simulink library "linearPlnt_ul"  (R2018a)
settings: Solver=VariableStepAuto  StartTime=0.0  StopTime=10.0  RelTol=1e-3
undefined symbols (not defined in the file): headingTimeConstant_s, maxSteadySpeed_mPs, speedTimeConstant_s
settings Model: Creator=mcobb  LastModifiedBy=mcobb

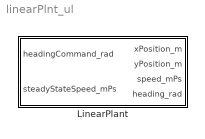
== system linearPlnt_ul ==
  LinearPlant : Subsystem

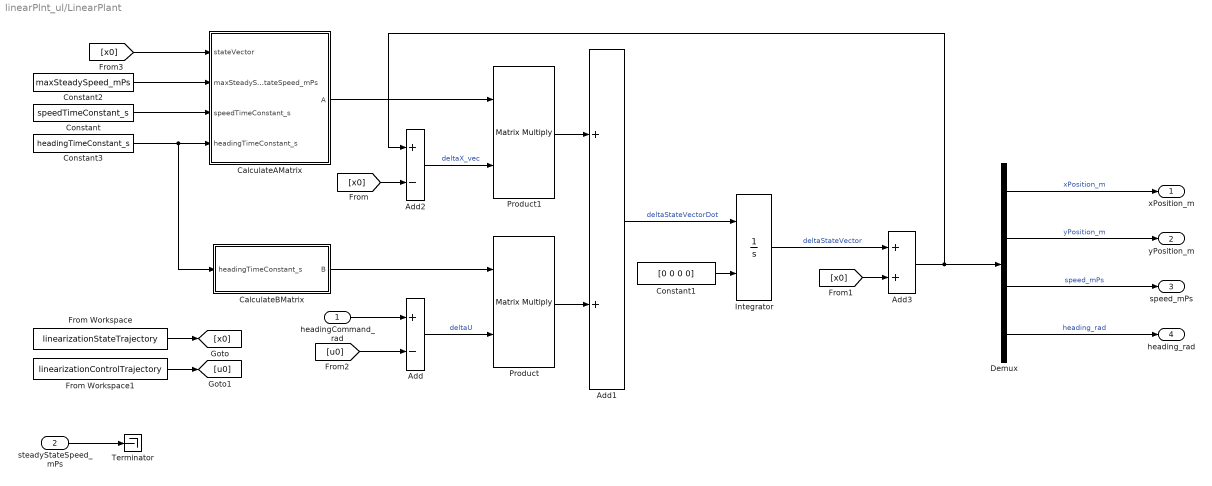
== system linearPlnt_ul/LinearPlant ==
  headingCommand_rad : Inport
  steadyStateSpeed_mPs : Inport  Port=2  PortDimensions=1
  Add : Sum  Inputs=+-
  Add1 : Sum
  Add2 : Sum  Inputs=+-
  Add3 : Sum
  CalculateAMatrix : MATLAB Function  TreatAsAtomicUnit=on
  CalculateBMatrix : MATLAB Function  TreatAsAtomicUnit=on
  Constant : Constant  Value=speedTimeConstant_s
  Constant1 : Constant  Value=[0 0 0 0]
  Constant2 : Constant  Value=maxSteadySpeed_mPs
  Constant3 : Constant  Value=headingTimeConstant_s
  Demux : Demux
  From Workspace : FromWorkspace  VariableName=linearizationStateTrajectory  SampleTime=0
  From Workspace1 : FromWorkspace  VariableName=linearizationControlTrajectory  SampleTime=0
  Integrator : Integrator  InitialConditionSource=external
  Product : Product  Multiplication=Matrix(*)
  Product1 : Product  Multiplication=Matrix(*)
  Terminator : Terminator
  xPosition_m : Outport
  yPosition_m : Outport  Port=2
  speed_mPs : Outport  Port=3
  heading_rad : Outport  Port=4
  wires:
  headingCommand_rad/1 -> Add/1
  Add/1 -> Product/2  "deltaU"
  Product/1 -> Add1/2
  Add2/1 -> Product1/2  "deltaX_vec"
  Add1/1 -> Integrator/1  "deltaStateVectorDot"
  Integrator/1 -> Add3/1  "deltaStateVector"
  Demux/1 -> xPosition_m/1  "xPosition_m"
  Demux/2 -> yPosition_m/1  "yPosition_m"
  Demux/3 -> speed_mPs/1  "speed_mPs"
  Demux/4 -> heading_rad/1  "heading_rad"
  Constant/1 -> CalculateAMatrix/3(speedTimeConstant_s)
  Constant3/1 -> CalculateBMatrix/1(headingTimeConstant_s), CalculateAMatrix/4(headingTimeConstant_s)
  CalculateBMatrix/1(B) -> Product/1
  CalculateAMatrix/1(A) -> Product1/1
  Product1/1 -> Add1/1
  From Workspace/1 -> [x0]
  [x0] -> Add2/2
  Add3/1 -> Add2/1, Demux/1
  [x0] -> Add3/2
  From Workspace1/1 -> [u0]
  [u0] -> Add/2
  Constant1/1 -> Integrator/2
  steadyStateSpeed_mPs/1 -> Terminator/1
  Constant2/1 -> CalculateAMatrix/2(maxSteadyStateSpeed_mPs)
  [x0] -> CalculateAMatrix/1(stateVector)

== matlab function linearPlnt_ul/LinearPlant/CalculateBMatrix ==
  data: headingTimeConstant_s input size=1; B output size=[4 1]
function B = fcn(headingTimeConstant_s)
B = [0 0 0 1/headingTimeConstant_s]';

== matlab function linearPlnt_ul/LinearPlant/CalculateAMatrix ==
  data: stateVector input size=[4 1]; A output size=[4 4]; maxSteadyStateSpeed_mPs input size=1; speedTimeConstant_s input; headingTimeConstant_s input size=1
function A = fcn(stateVector,maxSteadyStateSpeed_mPs,...
    speedTimeConstant_s,headingTimeConstant_s)
A = [...
    0 0  cos(stateVector(4))    -stateVector(3)*sin(stateVector(4));...
    0 0  sin(stateVector(4))     stateVector(3)*cos(stateVector(4));...
    0 0 -1/speedTimeConstant_s  -maxSteadyStateSpeed_mPs*sin(2*stateVector(4))/speedTimeConstant_s;...
    0 0 0                       -1/headingTimeConstant_s];
